simulink model "EPD_China_3_gen_With_Limitations"  (R2021b)
settings: Solver=VariableStepAuto  StartTime=0.0  StopTime=20  RelTol=1e-3
settings Model: Creator=vijay  LastModifiedBy=vijay

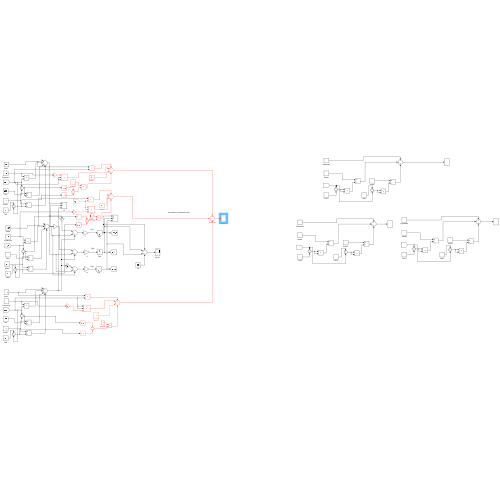
[thumbnail: Simulink's stored preview of the top-level diagram]
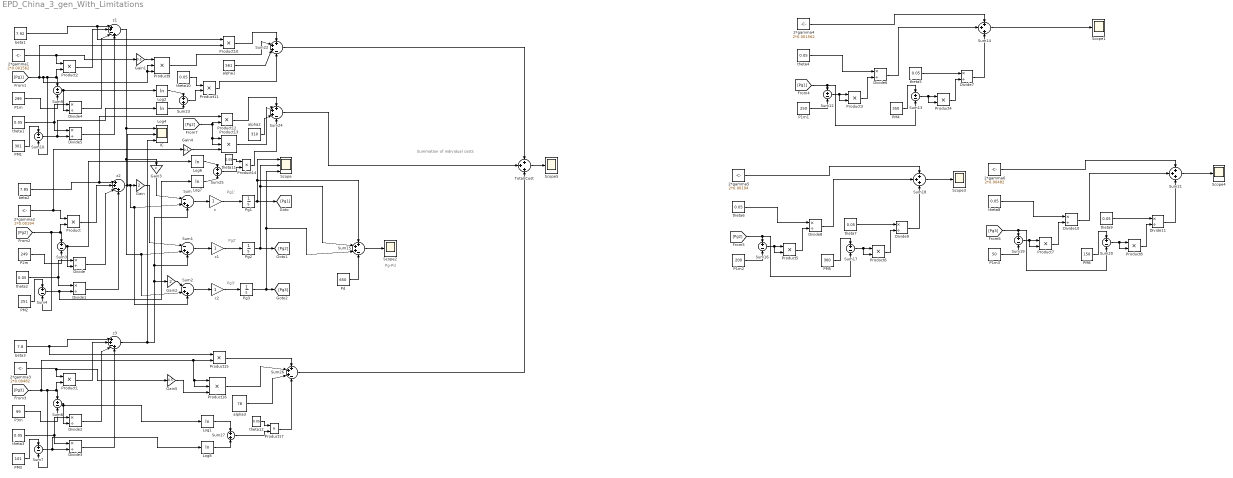
== system EPD_China_3_gen_With_Limitations ==
  note: Pg-Pd
  note: Summation of individual costs
  note: Pg3'
  note: Pg2'
  note: Pg1'
  2*gamma1 : Constant  Value=2*0.001562
  2*gamma2 : Constant  Value=2*0.00194
  2*gamma3 : Constant  Value=2*0.00482
  2*gamma4 : Constant  Value=2*0.001562
  2*gamma5 : Constant  Value=2*0.00194
  2*gamma6 : Constant  Value=2*0.00482
  Divide{,1..11} (12 alike) : Product  Inputs=*/
  Gain : Gain  Gain=2
  Gain1 : Gain  Gain=0.5
  Gain2 : Gain  Gain=2
  Gain3 : Gain  Gain=2
  Gain4 : Gain  Gain=0.5
  Gain5 : Gain  Gain=0.5
  IC : Scope  NumInputPorts=3
  Log{1..2,4,6..8} (6 alike) : Math  Operator=log  SignedPower=on  SaturateOnIntegerOverflow=on
  P1m : Constant  Value=299
  P1m1 : Constant  Value=250
  P1m2 : Constant  Value=200
  P1m3 : Constant  Value=50
  P2m : Constant  Value=249
  P3m : Constant  Value=99
  PM1 : Constant  Value=301
  PM2 : Constant  Value=251
  PM3 : Constant  Value=101
  PM4 : Constant  Value=350
  PM5 : Constant  Value=300
  PM6 : Constant  Value=150
  Pd : Constant  Value=650
  Pg1 : Integrator  InitialCondition=300
  Pg2 : Integrator  InitialCondition=250
  Pg3 : Integrator  InitialCondition=100
  Product{,1..8,10..12,14..15,17} (15 alike) : Product
  Product13 : Product  Inputs=3
  Product16 : Product  Inputs=3
  Product9 : Product  Inputs=3
  Scope : Scope  NumInputPorts=3
  Scope{1..5} (5 alike) : Scope
  Sum : Sum  Inputs=|-++
  Sum1 : Sum  Inputs=|-++
  Sum{3..4,6..7,9..10,12..13,16..17,19..20} (12 alike) : Sum  Inputs=+-
  Sum14 : Sum  Inputs=+++
  Sum{15,22,24,26} (4 alike) : Sum  Inputs=+++-
  Sum18 : Sum  Inputs=+++
  Sum2 : Sum  Inputs=|-++
  Sum21 : Sum  Inputs=+++
  Sum23 : Sum
  Sum25 : Sum
  Sum27 : Sum
  Total Cost : Sum  Inputs=+++
  alpha1 : Constant  Value=561
  alpha2 : Constant  Value=310
  alpha3 : Constant  Value=78
  beta1 : Constant  Value=7.92
  beta2 : Constant  Value=7.85
  beta3 : Constant  Value=7.8
  c : Gain
  c1 : Gain
  c2 : Gain
  theta{1..12} (12 alike) : Constant  Value=0.05
  z1 : Sum  Inputs=|++-+
  z2 : Sum  Inputs=|++-+
  z3 : Sum  Inputs=|++-+
  wires:
  Sum/1 -> c/1
  c/1 -> Pg1/1
  Pg1/1 -> Sum15/1, Scope/1, [Pg1]
  Sum1/1 -> c1/1
  c1/1 -> Pg2/1
  Pg2/1 -> Sum15/2, Scope/2, [Pg2]
  Sum2/1 -> c2/1
  c2/1 -> Pg3/1
  Pg3/1 -> Sum15/3, Scope/3, [Pg3]
  2*gamma2/1 -> Gain4/1, Product/1
  [Pg2] -> Sum4/2, Sum3/1, Product/2
  P2m/1 -> Sum3/2
  theta2/1 -> Divide1/1, Divide/1
  Sum3/1 -> Log6/1, Divide/2
  PM2/1 -> Sum4/1
  Sum4/1 -> Log7/1, Divide1/2
  beta2/1 -> Product12/1, z2/1
  Product/1 -> z2/2
  Divide/1 -> z2/3
  Divide1/1 -> z2/4
  z2/1 -> IC/2, Sum2/3, Sum/2, Gain/1
  beta3/1 -> Product15/1, z3/1
  Product1/1 -> z3/2
  Sum7/1 -> Log8/1, Divide3/2
  z3/1 -> Gain2/1, Sum1/3, Sum/3, IC/3
  Sum6/1 -> Log1/1, Divide2/2
  P3m/1 -> Sum6/2
  theta3/1 -> Divide3/1, Divide2/1
  [Pg3] -> Product16/2, Product16/1, Product15/2, Sum7/2, Sum6/1, Product1/2
  2*gamma3/1 -> Gain5/1, Product1/1
  PM3/1 -> Sum7/1
  Divide3/1 -> z3/4
  Divide2/1 -> z3/3
  [Pg1] -> Product10/2, Product9/3, Product9/2, Sum10/2, Sum9/1, Product2/2
  2*gamma1/1 -> Gain1/1, Product2/1
  Sum9/1 -> Log2/1, Divide4/2
  Sum10/1 -> Log4/1, Divide5/2
  beta1/1 -> Product10/1, z1/1
  PM1/1 -> Sum10/1
  theta1/1 -> Divide5/1, Divide4/1
  Divide4/1 -> z1/3
  Divide5/1 -> z1/4
  Product2/1 -> z1/2
  P1m/1 -> Sum9/2
  Gain3/1 -> Sum/1
  z1/1 -> Gain3/1, Sum2/2, Sum1/2, IC/1
  Gain/1 -> Sum1/1
  Gain2/1 -> Sum2/1
  [Pg1] -> Sum13/2, Sum12/1
  P1m1/1 -> Sum12/2
  Sum12/1 -> Product3/2, Product3/1
  theta4/1 -> Divide6/1
  Product3/1 -> Divide6/2
  PM4/1 -> Sum13/1
  Sum13/1 -> Product4/2, Product4/1
  theta5/1 -> Divide7/1
  Product4/1 -> Divide7/2
  Divide7/1 -> Sum14/3
  Divide6/1 -> Sum14/2
  2*gamma4/1 -> Sum14/1
  Sum14/1 -> Scope1/1
  Pd/1 -> Sum15/4
  Sum15/1 -> Scope2/1
  Sum17/1 -> Product6/2, Product6/1
  2*gamma5/1 -> Sum18/1
  Product6/1 -> Divide9/2
  Sum16/1 -> Product5/2, Product5/1
  Divide9/1 -> Sum18/3
  [Pg2] -> Sum17/2, Sum16/1
  PM5/1 -> Sum17/1
  theta7/1 -> Divide9/1
  P1m2/1 -> Sum16/2
  Divide8/1 -> Sum18/2
  Product5/1 -> Divide8/2
  theta6/1 -> Divide8/1
  Sum20/1 -> Product8/2, Product8/1
  2*gamma6/1 -> Sum21/1
  Product8/1 -> Divide11/2
  Sum19/1 -> Product7/2, Product7/1
  Divide11/1 -> Sum21/3
  [Pg3] -> Sum20/2, Sum19/1
  PM6/1 -> Sum20/1
  theta9/1 -> Divide11/1
  P1m3/1 -> Sum19/2
  Divide10/1 -> Sum21/2
  Product7/1 -> Divide10/2
  theta8/1 -> Divide10/1
  Sum18/1 -> Scope3/1
  Sum21/1 -> Scope4/1
  Gain1/1 -> Product9/1
  Product10/1 -> Sum22/1
  Product9/1 -> Sum22/2
  alpha1/1 -> Sum22/3
  Log2/1 -> Sum23/1
  Log4/1 -> Sum23/2
  theta10/1 -> Product11/1
  Sum23/1 -> Product11/2
  Product11/1 -> Sum22/4
  [Pg2] -> Product13/2, Product13/1, Product12/2
  Gain4/1 -> Product13/3
  Product12/1 -> Sum24/1
  Product13/1 -> Sum24/2
  alpha2/1 -> Sum24/3
  Log6/1 -> Sum25/1
  Log7/1 -> Sum25/2
  Sum25/1 -> Product14/2
  theta11/1 -> Product14/1
  Product14/1 -> Sum24/4
  Gain5/1 -> Product16/3
  Product15/1 -> Sum26/1
  Product16/1 -> Sum26/2
  alpha3/1 -> Sum26/3
  Log1/1 -> Sum27/1
  Log8/1 -> Sum27/2
  theta12/1 -> Product17/1
  Sum27/1 -> Product17/2
  Product17/1 -> Sum26/4
  Sum24/1 -> Total Cost/2
  Sum22/1 -> Total Cost/1
  Sum26/1 -> Total Cost/3
  Total Cost/1 -> Scope5/1
